simulink model "sampleModel219"  (R2021b)
settings: Solver=VariableStepAuto  StartTime=0.0  StopTime=10.0  RelTol=1e-3
undefined symbols (not defined in the file or in its folder): Newton, Raphson
libraries: simulink x10, slpidlib x1
settings Model: Creator=user  LastModifiedBy=user

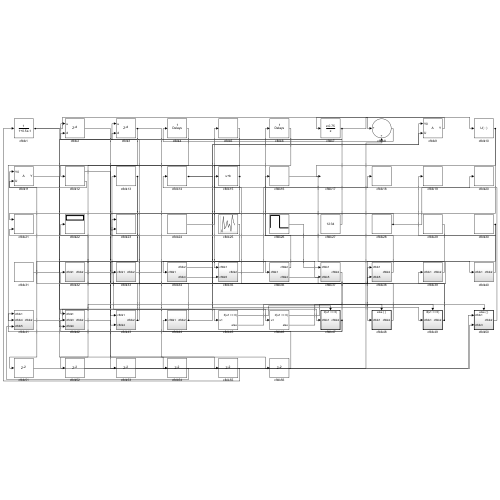
[thumbnail: Simulink's stored preview of the top-level diagram]
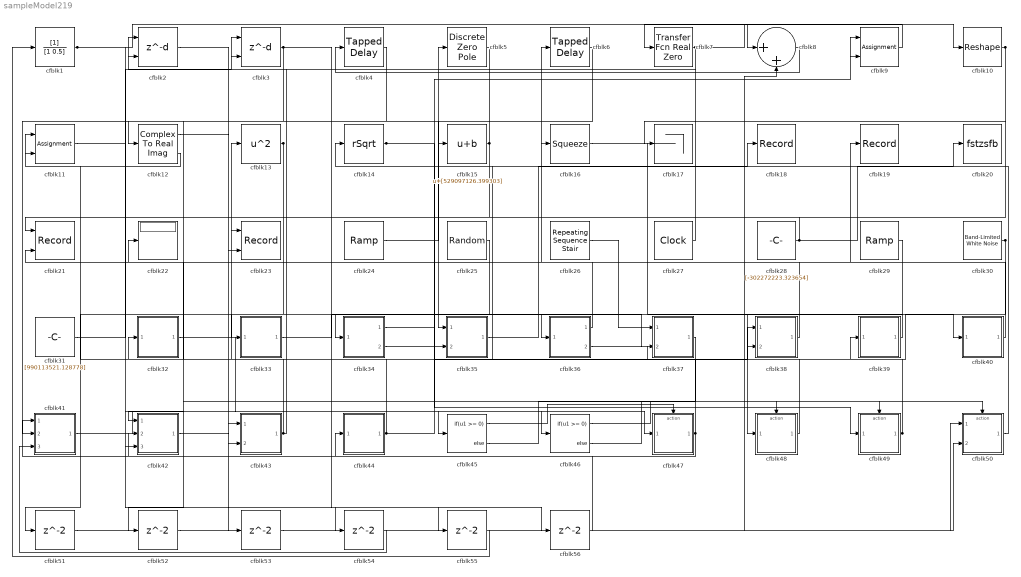
== system sampleModel219 ==
  cfblk1 : DiscreteFilter  SampleTime=1
  cfblk10 : Reshape
  cfblk11 : Assignment  DiagnosticForDimensions=Warning  IndexOptions=Index vector (dialog)  Indices=1  OutputSizes=1
  cfblk12 : ComplexToRealImag
  cfblk13 : Math  Operator=square  SaturateOnIntegerOverflow=on
  cfblk14 : Sqrt  Operator=rSqrt  AlgorithmType=Newton-Raphson  SaturateOnIntegerOverflow=on
  cfblk15 : Bias  Bias=[529097126.399303]
  cfblk16 : Squeeze
  cfblk17 : Terminator
  cfblk18 : Record  FileSettingsInternal="{\"entries\":[{\"content\":{\"excelSettings\":{\"content\":{},\"type\":\"Streamout.ExcelSettings\"}},\"type\":\"Streamout.FileSettingStorage\",\"uuid\":\"844487d7-c96f-4e93-af2b-bf0dbd47c6b0\"}],\"packageUris\":[\"http://schema.mathworks.com/mf0/streamout_blocks/R2020a\"],\"version\":\"1.0\"}"  SignalsInternal="{\"entries\":[{\"content\":{\"signals\":[{\"content\":{\"blockPath\":[\"sampleModel219/cfblk18\"],\"channel\":[],\"dimensions\":[1],\"domain\":\"sampleModel219/cfblk18\",\"lineColor\":\"#22b573\",\"plots\":[1],\"port\":1,\"sid\":[\"\"],\"signalID\":8491,\"signalName\":\"cfblk35\"},\"type\":\"RecordBlkView.Signal\",\"uuid\":\"787874c2-7397-4e25-ab33-5eaf260bd77f\"}]},\"type\":\"RecordBlkView.InputSignals\",\"uuid\":\"995c5a30-6b30-4493-8084-ea241034027c\"}],\"packageUris\":[\"http://schema.mathworks.com/mf0/streamout_blocks/R2020a\"],\"version\":\"1.0\"}"  VisualizationBindings="{\"sparklinesplugin\":{\"info\":[{\"bindingParametersList\":[],\"subplotID\":1}]}}"
  cfblk19 : Record  FileSettingsInternal="{\"entries\":[{\"content\":{\"excelSettings\":{\"content\":{},\"type\":\"Streamout.ExcelSettings\"}},\"type\":\"Streamout.FileSettingStorage\",\"uuid\":\"375c4ac3-81d9-474c-aef5-ac18971b0f9f\"}],\"packageUris\":[\"http://schema.mathworks.com/mf0/streamout_blocks/R2020a\"],\"version\":\"1.0\"}"  SignalsInternal="{\"entries\":[{\"content\":{\"signals\":[{\"content\":{\"blockPath\":[\"sampleModel219/cfblk19\"],\"channel\":[],\"dimensions\":[1],\"domain\":\"sampleModel219/cfblk19\",\"lineColor\":\"#0072bd\",\"plots\":[1],\"port\":1,\"sid\":[\"\"],\"signalID\":8495,\"signalName\":\"cfblk40\"},\"type\":\"RecordBlkView.Signal\",\"uuid\":\"74e9c32f-e3b0-48a6-9fbb-b049483dea16\"}]},\"type\":\"RecordBlkView.InputSignals\",\"uuid\":\"63b3f7b2-6be4-4c98-a56e-562f848dcaa4\"}],\"packageUris\":[\"http://schema.mathworks.com/mf0/streamout_blocks/R2020a\"],\"version\":\"1.0\"}"  VisualizationBindings="{\"sparklinesplugin\":{\"info\":[{\"bindingParametersList\":[],\"subplotID\":1}]}}"
  cfblk2 : Delay  DelayLengthSource=Input port  SampleTime=1
      settings: InputPortMap=u0,p1
  cfblk20 : ToWorkspace  VariableName=fstzsfb  SaveFormat=Timeseries  SampleTime=-1
  cfblk21 : Record  FileSettingsInternal="{\"entries\":[{\"content\":{\"excelSettings\":{\"content\":{},\"type\":\"Streamout.ExcelSettings\"}},\"type\":\"Streamout.FileSettingStorage\",\"uuid\":\"16af1733-4450-4020-9d88-b2d3b491021f\"}],\"packageUris\":[\"http://schema.mathworks.com/mf0/streamout_blocks/R2020a\"],\"version\":\"1.0\"}"  Layout=[1 1]  SignalsInternal="{\"entries\":[{\"content\":{\"signals\":[{\"content\":{\"blockPath\":[\"sampleModel219/cfblk21\"],\"channel\":[],\"dimensions\":[1],\"domain\":\"sampleModel219/cfblk21\",\"lineColor\":\"#a2142f\",\"plots\":[1],\"port\":1,\"sid\":[\"\"],\"signalID\":8475,\"signalName\":\"cfblk28\"},\"type\":\"RecordBlkView.Signal\",\"uuid\":\"d653b768-9833-42c3-a752-d42a356465da\"},{\"content\":{\"blockPath\":[\"sampleModel219/cfblk21\"],\"channel\":[],\"dimensions\":[1],\"domain\":\"sampleModel219/cfblk21\",\"lineColor\":\"#139fff\",\"plots\":[1],\"port\":2,\"sid\":[\"\"],\"signalID\":8479,\"signalName\":\"cfblk30\"},\"type\":\"RecordBlkView.Signal\",\"uuid\":\"69c004cc-b0a6-4d74-83ed-d32cbb778e8f\"}]},\"type\":\"RecordBlkView.InputSignals\",\"uuid\":\"59e627b1-992e-4978-a83e-8969309c215d\"}],\"packageUris\":[\"http://schema.mathworks.com/mf0/streamout_blocks/R2020a\"],\"version\":\"1.0\"}"  VisualizationBindings="{\"xyplotplugin\":{\"info\":[{\"series\":[{\"bindingParametersList\":[{\"parameter\":\"X-Axis\",\"signalID\":8475,\"signalName\":\"cfblk28\"},{\"parameter\":\"Y-Axis\",\"signalID\":8479,\"signalName\":\"cfblk30\"}],\"seriesID\":18144}],\"subplotID\":1}]}}"  CompatibilityTag=XY
  cfblk22 : Display
  cfblk23 : Record  FileSettingsInternal="{\"entries\":[{\"content\":{\"excelSettings\":{\"content\":{},\"type\":\"Streamout.ExcelSettings\"}},\"type\":\"Streamout.FileSettingStorage\",\"uuid\":\"9a815e8d-0a58-4833-81d0-cb5a31f32881\"}],\"packageUris\":[\"http://schema.mathworks.com/mf0/streamout_blocks/R2020a\"],\"version\":\"1.0\"}"  Layout=[1 1]  SignalsInternal="{\"entries\":[{\"content\":{\"signals\":[{\"content\":{\"blockPath\":[\"sampleModel219/cfblk23\"],\"channel\":[],\"dimensions\":[1],\"domain\":\"sampleModel219/cfblk23\",\"lineColor\":\"#a2142f\",\"plots\":[1],\"port\":1,\"sid\":[\"\"],\"signalID\":8483,\"signalName\":\"cfblk43\"},\"type\":\"RecordBlkView.Signal\",\"uuid\":\"355acc69-8332-465b-8783-850e357cb4b5\"},{\"content\":{\"blockPath\":[\"sampleModel219/cfblk23\"],\"channel\":[],\"dimensions\":[1],\"domain\":\"sampleModel219/cfblk23\",\"lineColor\":\"#139fff\",\"plots\":[1],\"port\":2,\"sid\":[\"\"],\"signalID\":8487,\"signalName\":\"cfblk3\"},\"type\":\"RecordBlkView.Signal\",\"uuid\":\"6b89a9b7-5837-4694-8f1f-2255a32fdfec\"}]},\"type\":\"RecordBlkView.InputSignals\",\"uuid\":\"31b18c4c-20c7-4640-a172-71e28492e71b\"}],\"packageUris\":[\"http://schema.mathworks.com/mf0/streamout_blocks/R2020a\"],\"version\":\"1.0\"}"  VisualizationBindings="{\"xyplotplugin\":{\"info\":[{\"series\":[{\"bindingParametersList\":[{\"parameter\":\"X-Axis\",\"signalID\":8483,\"signalName\":\"cfblk43\"},{\"parameter\":\"Y-Axis\",\"signalID\":8487,\"signalName\":\"cfblk3\"}],\"seriesID\":58549}],\"subplotID\":1}]}}"  CompatibilityTag=XY
  cfblk24 : simulink/Sources/Ramp  slope=[538.350002]  start=[35.034303]  InitialOutput=[175020.795181]
  cfblk25 : UniformRandomNumber  Minimum=[-4191822465.297766]  Maximum=[714476580.782402]  Seed=[94825884.000000]  SampleTime=0.1
  cfblk26 : simulink/Sources/Repeating Sequence Stair  OutValues=[713740107.884745, 662895871.123101]  tsamp=-1  OutMin=[]  OutMax=[]  OutDataTypeStr=double  OutputDataTypeScalingMode=double  OutDataType=fixdt(0,8)  ConRadixGroup=Best Precision: Vector-wise  OutScaling=2^-12
  cfblk27 : DigitalClock
  cfblk28 : Constant  Value=[-302272223.323654]  SampleTime=1
  cfblk29 : simulink/Sources/Ramp  slope=[-6066.908526]  start=[12.864614]  InitialOutput=[-357193.719441]
  cfblk3 : Delay  DelayLengthSource=Input port  SampleTime=1
      settings: InputPortMap=u0,p1
  cfblk30 : simulink/Sources/Band-Limited White Noise  Cov=[1010731546.581772]  Ts=0.1  seed=[7249196664.000000]
  cfblk31 : Constant  Value=[990113521.128778]  SampleTime=1
  cfblk32 : Subsystem
  cfblk33 : Subsystem
  cfblk34 : Subsystem
  cfblk35 : Subsystem
  cfblk36 : Subsystem
  cfblk37 : Subsystem
  cfblk38 : Subsystem
  cfblk39 : Subsystem
  cfblk4 : simulink/Discrete/Tapped Delay  vinit=0.0  samptime=-1  NumDelays=1  DelayOrder=Oldest  includeCurrent=off
  cfblk40 : Subsystem
  cfblk41 : Subsystem
  cfblk42 : Subsystem
  cfblk43 : Subsystem
  cfblk44 : Subsystem
  cfblk45 : If  IfExpression=u1 >= 0  SampleTime=1
  cfblk46 : If  IfExpression=u1 >= 0  SampleTime=1
  cfblk47 : Subsystem  TreatAsAtomicUnit=on
  cfblk48 : Subsystem  TreatAsAtomicUnit=on
  cfblk49 : Subsystem  TreatAsAtomicUnit=on
  cfblk5 : DiscreteZeroPole  Poles=[0 0.5]  Gain=1
  cfblk50 : Subsystem  TreatAsAtomicUnit=on
  cfblk{51..56} (6 alike) : Delay  SampleTime=1
  cfblk6 : simulink/Discrete/Tapped Delay  vinit=0.0  samptime=-1  NumDelays=1  DelayOrder=Oldest  includeCurrent=off
  cfblk7 : simulink/Discrete/Transfer Fcn Real Zero  ZeroZ=0.75  ICPrevInput=0.0  DoSatur=off
      settings: SourceProductBaseCode=SL
  cfblk8 : Sum  Inputs=|++
  cfblk9 : Assignment  DiagnosticForDimensions=Warning  IndexOptions=Index vector (dialog)  Indices=1  OutputSizes=1
  wires:
  cfblk15/1 -> cfblk12/1, cfblk43/2(cfblk4)
  cfblk1/1 -> cfblk8/1, cfblk47/1(cfblk1)
  cfblk29/1 -> cfblk48/1(cfblk1)
  cfblk30/1 -> cfblk39/1(cfblk1), cfblk21/2
  cfblk50/1(cfblk2) -> cfblk14/1
  cfblk41/1(cfblk2) -> cfblk45/1
  cfblk16/1 -> cfblk40/1(cfblk1)
  cfblk43/1(cfblk2) -> cfblk13/1, cfblk23/1
  cfblk26/1 -> cfblk37/1(cfblk1)
  cfblk32/1(cfblk2) -> cfblk46/1
  cfblk39/1(cfblk2) -> cfblk33/1(cfblk1)
  cfblk44/1(cfblk2) -> cfblk32/1(cfblk1), cfblk9/1
  cfblk25/1 -> cfblk34/1(cfblk1)
  cfblk8/1 -> cfblk4/1
  cfblk36/1(cfblk2) -> cfblk6/1
  cfblk9/1 -> cfblk7/1
  cfblk31/1 -> cfblk3/1
  cfblk27/1 -> cfblk2/1
  cfblk40/1(cfblk2) -> cfblk19/1
  cfblk47/1(cfblk2) -> cfblk22/1, cfblk44/1(cfblk1), cfblk42/2(cfblk3)
  cfblk33/1(cfblk2) -> cfblk36/1(cfblk1)
  cfblk24/1 -> cfblk5/1
  cfblk28/1 -> cfblk21/1, cfblk20/1
  cfblk5/1 -> cfblk35/1(cfblk1)
  cfblk48/1(cfblk2) -> cfblk3/2
  cfblk10/1 -> cfblk35/2(cfblk5), cfblk17/1
  cfblk7/1 -> cfblk2/2, cfblk10/1
  cfblk3/1 -> cfblk23/2, cfblk56/1
  cfblk38/1(cfblk2) -> cfblk16/1
  cfblk36/2(cfblk4) -> cfblk38/1(cfblk1)
  cfblk4/1 -> cfblk41/2(cfblk4)
  cfblk13/1 -> cfblk42/3(cfblk4), cfblk51/1
  cfblk49/1(cfblk2) -> cfblk15/1, cfblk11/2
  cfblk35/1(cfblk2) -> cfblk18/1
  cfblk14/1 -> cfblk37/2(cfblk5), cfblk9/2
  cfblk34/1(cfblk2) -> cfblk49/1(cfblk1)
  cfblk34/2(cfblk4) -> cfblk38/2(cfblk5)
  cfblk12/1 -> cfblk43/1(cfblk1)
  cfblk12/2 -> cfblk11/1
  cfblk6/1 -> cfblk42/1(cfblk1)
  cfblk45/1 -> cfblk47/Action
  cfblk45/2 -> cfblk48/Action
  cfblk46/1 -> cfblk49/Action
  cfblk46/2 -> cfblk50/Action
  cfblk51/1 -> cfblk50/2(cfblk3)
  cfblk37/1(cfblk2) -> cfblk52/1
  cfblk52/1 -> cfblk8/2
  cfblk2/1 -> cfblk53/1
  cfblk53/1 -> cfblk50/1(cfblk1)
  cfblk42/1(cfblk2) -> cfblk54/1
  cfblk54/1 -> cfblk41/3(cfblk5)
  cfblk11/1 -> cfblk55/1
  cfblk55/1 -> cfblk1/1
  cfblk56/1 -> cfblk41/1(cfblk1)

== system sampleModel219/cfblk32 ==
  cfblk1 : Inport
  cfblk3 : Signum
  cfblk2 : Outport
  wires:
  cfblk1/1 -> cfblk2/1, cfblk3/1

== system sampleModel219/cfblk33 ==
  cfblk1 : Inport
  cfblk3 : ComplexToRealImag
  cfblk2 : Outport
  wires:
  cfblk1/1 -> cfblk3/1
  cfblk3/1 -> cfblk2/1

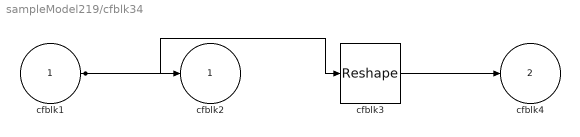
== system sampleModel219/cfblk34 ==
  cfblk1 : Inport
  cfblk3 : Reshape
  cfblk2 : Outport
  cfblk4 : Outport  Port=2
  wires:
  cfblk1/1 -> cfblk2/1, cfblk3/1
  cfblk3/1 -> cfblk4/1

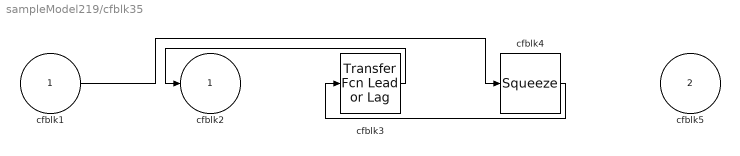
== system sampleModel219/cfblk35 ==
  cfblk1 : Inport
  cfblk5 : Inport  Port=2
  cfblk3 : simulink/Discrete/Transfer Fcn Lead or Lag  PoleZ=0.95  ZeroZ=0.75  ICPrevOutput=0.0  ICPrevInput=0.0  DoSatur=off
      settings: SourceProductBaseCode=SL
  cfblk4 : Squeeze
  cfblk2 : Outport
  wires:
  cfblk3/1 -> cfblk2/1
  cfblk4/1 -> cfblk3/1
  cfblk1/1 -> cfblk4/1

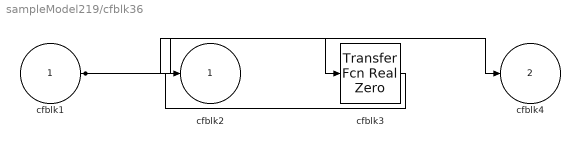
== system sampleModel219/cfblk36 ==
  cfblk1 : Inport
  cfblk3 : simulink/Discrete/Transfer Fcn Real Zero  ZeroZ=0.75  ICPrevInput=0.0  DoSatur=off
      settings: SourceProductBaseCode=SL
  cfblk2 : Outport
  cfblk4 : Outport  Port=2
  wires:
  cfblk1/1 -> cfblk3/1, cfblk4/1
  cfblk3/1 -> cfblk2/1

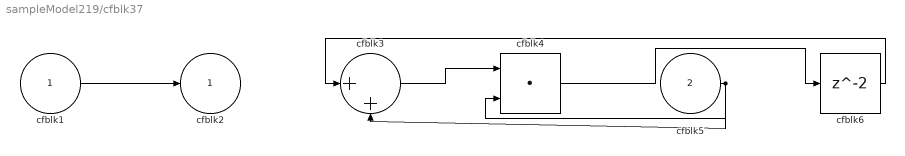
== system sampleModel219/cfblk37 ==
  cfblk1 : Inport
  cfblk5 : Inport  Port=2
  cfblk3 : Sum  Inputs=|++
  cfblk4 : DotProduct  InputSameDT=on  OutDataTypeStr=Inherit: Inherit via internal rule
  cfblk6 : Delay  SampleTime=1
  cfblk2 : Outport
  wires:
  cfblk1/1 -> cfblk2/1
  cfblk5/1 -> cfblk3/2, cfblk4/2
  cfblk3/1 -> cfblk4/1
  cfblk4/1 -> cfblk6/1
  cfblk6/1 -> cfblk3/1

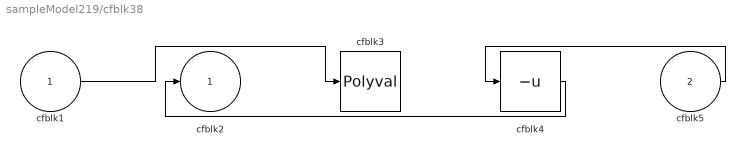
== system sampleModel219/cfblk38 ==
  cfblk1 : Inport
  cfblk5 : Inport  Port=2
  cfblk3 : Polyval  Coefs=[ +2.081618890e-019, -1.441693666e-014, +4.719686976e-010, -8.536869453e-006, +1.621573104e-001, -8.087801117e+001 ]
  cfblk4 : UnaryMinus
  cfblk2 : Outport
  wires:
  cfblk5/1 -> cfblk4/1
  cfblk4/1 -> cfblk2/1
  cfblk1/1 -> cfblk3/1

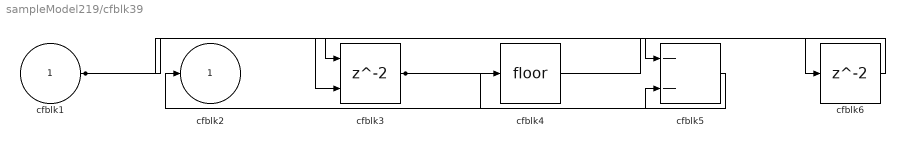
== system sampleModel219/cfblk39 ==
  cfblk1 : Inport
  cfblk3 : Delay  ShowEnablePort=on  SampleTime=1
      settings: InputPortMap=u0,e6
  cfblk4 : Rounding
  cfblk5 : Sum  Inputs=--
  cfblk6 : Delay  SampleTime=1
  cfblk2 : Outport
  wires:
  cfblk3/1 -> cfblk4/1, cfblk5/2
  cfblk5/1 -> cfblk2/1
  cfblk1/1 -> cfblk3/2, cfblk5/1
  cfblk4/1 -> cfblk6/1
  cfblk6/1 -> cfblk3/1

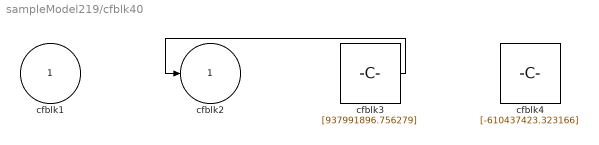
== system sampleModel219/cfblk40 ==
  cfblk1 : Inport
  cfblk3 : Constant  Value=[937991896.756279]  SampleTime=1
  cfblk4 : Constant  Value=[-610437423.323166]  SampleTime=1
  cfblk2 : Outport
  wires:
  cfblk3/1 -> cfblk2/1

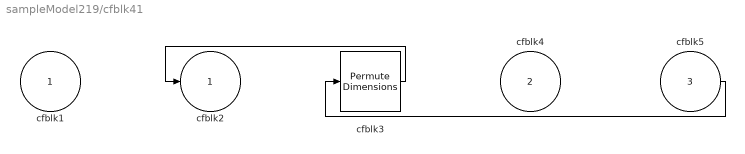
== system sampleModel219/cfblk41 ==
  cfblk1 : Inport
  cfblk4 : Inport  Port=2
  cfblk5 : Inport  Port=3
  cfblk3 : PermuteDimensions
  cfblk2 : Outport
  wires:
  cfblk3/1 -> cfblk2/1
  cfblk5/1 -> cfblk3/1

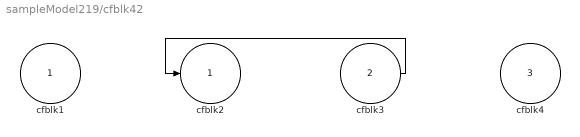
== system sampleModel219/cfblk42 ==
  cfblk1 : Inport
  cfblk3 : Inport  Port=2
  cfblk4 : Inport  Port=3
  cfblk2 : Outport
  wires:
  cfblk3/1 -> cfblk2/1

== system sampleModel219/cfblk43 ==
  cfblk1 : Inport
  cfblk4 : Inport  Port=2
  cfblk3 : Assignment  DiagnosticForDimensions=Warning  IndexOptions=Index vector (dialog)  Indices=1  OutputSizes=1
  cfblk2 : Outport
  wires:
  cfblk3/1 -> cfblk2/1
  cfblk4/1 -> cfblk3/1
  cfblk1/1 -> cfblk3/2

== system sampleModel219/cfblk44 ==
  cfblk1 : Inport
  cfblk3 : DiscreteTransferFcn  SampleTime=1
  cfblk2 : Outport
  wires:
  cfblk3/1 -> cfblk2/1
  cfblk1/1 -> cfblk3/1

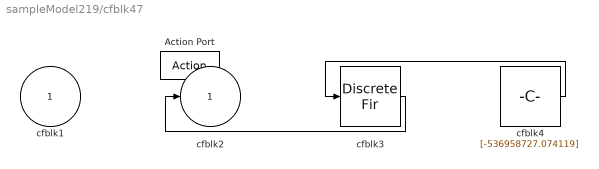
== system sampleModel219/cfblk47 ==
  cfblk1 : Inport
  Action Port : ActionPort  ActionPortLabel=if(u1 >= 0)
  cfblk3 : DiscreteFir
  cfblk4 : Constant  Value=[-536958727.074119]  SampleTime=1
  cfblk2 : Outport
  wires:
  cfblk4/1 -> cfblk3/1
  cfblk3/1 -> cfblk2/1

== system sampleModel219/cfblk48 ==
  cfblk1 : Inport
  Action Port : ActionPort  ActionPortLabel=else
  cfblk3 : slpidlib/PID Controller  Controller=PID  Form=Parallel  TimeDomain=Discrete-time  UseExternalTs=off  SampleTime=-1  IntegratorMethod=Forward Euler  FilterMethod=Forward Euler  ControllerParametersSource=internal  P=1  I=1  D=0  UseFilter=on  N=100  TunerSelectOption=Transfer Function Based (PID Tuner App)  InitialConditionSource=internal  InitialConditionForIntegrator=0  InitialConditionForFilter=0  DifferentiatorICPrevScaledInput=0  ExternalReset=none  TrackingMode=off  Kt=1  LimitOutput=off  SatLimitsSource=internal  UpperSaturationLimit=inf  LowerSaturationLimit=-inf  LinearizeAsGain=off  AntiWindupMode=none  Kb=1  POutMin=[]  POutMax=[]  IOutMin=[]  IOutMax=[]  DOutMin=[]  DOutMax=[]  NOutMin=[]  NOutMax=[]  SumOutMin=[]  SumOutMax=[]  SaturationOutMin=[]  SaturationOutMax=[]  PParamMin=[]  PParamMax=[]  IParamMin=[]  IParamMax=[]  DParamMin=[]  DParamMax=[]  NParamMin=[]  NParamMax=[]  KbParamMin=[]  KbParamMax=[]  KtParamMin=[]  KtParamMax=[]  KbOutMin=[]  KbOutMax=[]  KtOutMin=[]  KtOutMax=[]  IntegratorOutMin=[]  IntegratorOutMax=[]  FilterOutMin=[]  FilterOutMax=[]  SumI1OutMin=[]  SumI1OutMax=[]  SumI2OutMin=[]  SumI2OutMax=[]  SumI3OutMin=[]  SumI3OutMax=[]  SumI4OutMin=[]  SumI4OutMax=[]  SumDOutMin=[]  SumDOutMax=[]  DifferentiatorOutMin=[]  DifferentiatorOutMax=[]  FilterDiffOutCoefMin=[]  FilterDiffOutCoefMax=[]  ReciprocalOutMin=[]  ReciprocalOutMax=[]  SumDenOutMin=[]  SumDenOutMax=[]  SumNumOutMin=[]  SumNumOutMax=[]  DivideOutMin=[]  DivideOutMax=[]  UdiffTsProdOutMin=[]  UdiffTsProdOutMax=[]  NTsProdOutMin=[]  NTsProdOutMax=[]  UintegralTsProdOutMin=[]  UintegralTsProdOutMax=[]  UngainTsProdOutMin=[]  UngainTsProdOutMax=[]  IntegratorContinuousStateAttributes=''  IntegratorStateMustResolveToSignalObject=off  IntegratorRTWStateStorageClass=Auto  FilterContinuousStateAttributes=''  FilterStateMustResolveToSignalObject=off  FilterRTWStateStorageClass=Auto  ParallelPVariant=InternalParameters  IdealPVariant=Disabled  IVariant=InternalParameters  DVariant=InternalParameters  IntegratorVariant=Discrete  SatVariant=Disabled  AWVariant=Passthrough  PCopyVariant=Disabled  TRVariant=Disabled  FdbkBlocksVariant=Forward  IdealPFdbkVariant=Disabled  SatFdbkVariant=Disabled  DerivativeFilterVariant=ForwardEulerFilter  NVariant=InternalParameters  NCopyVariant=Disabled  FilterICVariant=InternalICsFilter  IntegratorICVariant=InternalICs  ExternalResetVariant=Disabled  TRSumVariant=Passthrough  SumFdbkVariant=Disabled  SumVariant=Sum_PID  TsampFilterVariant=InternalTs  TsampNgainVariant=Passthrough  TsampIntegralVariant=Passthrough  ExternalSaturationOutDataTypeStr=Inherit: Same as second input
  cfblk2 : Outport
  wires:
  cfblk1/1 -> cfblk3/1
  cfblk3/1 -> cfblk2/1

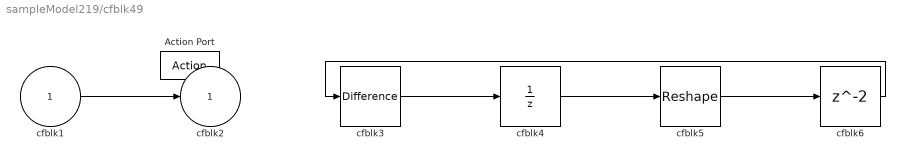
== system sampleModel219/cfblk49 ==
  cfblk1 : Inport
  Action Port : ActionPort  ActionPortLabel=if(u1 >= 0)
  cfblk3 : simulink/Discrete/Difference  ICPrevInput=0.0  OutMin=[]  OutMax=[]  OutDataTypeStr=Inherit: Inherit via back propagation  OutDataType=fixdt(1, 16)  OutScaling=2^-10  DoSatur=off
  cfblk4 : UnitDelay  SampleTime=-1  HasFrameUpgradeWarning=on
  cfblk5 : Reshape
  cfblk6 : Delay
  cfblk2 : Outport
  wires:
  cfblk1/1 -> cfblk2/1
  cfblk4/1 -> cfblk5/1
  cfblk3/1 -> cfblk4/1
  cfblk5/1 -> cfblk6/1
  cfblk6/1 -> cfblk3/1

== system sampleModel219/cfblk50 ==
  cfblk1 : Inport
  cfblk3 : Inport  Port=2
  Action Port : ActionPort  ActionPortLabel=else
  cfblk2 : Outport
  wires:
  cfblk3/1 -> cfblk2/1
